simulink model "sim_punto4"  (R2021b)
settings: Solver=VariableStepAuto  StartTime=0.0  StopTime=10.0  RelTol=1e-3
values from neighbouring files (symbols this model uses):
  A = [0 1 0 0 0 0 0 0 0 0 0 0 ... (first row only)    [punto4.m]
  B = [0; 0; 0; 0; 0; 0; 0; 0; 0; 0; 0; 1]    [punto4.m]
  C = [1 0 0 0 0 0 0 0 0 0 0 0]    [punto4.m]
  C_states = eye(12)    [punto4.m]
  D_states = [0 0 0 0 0 0 0 0 0 0 0 0]'    [punto4.m]
  N3 = 27    [punto4.m]
  Q = [1+q 0 0 0 0 0 0 0 0 0 0 0 ... (first row only)    [punto4.m]
  R = r    (= 1e-05)    [punto4.m]
  S = [0 0 0 0 0 0 0 0 0 0 0 0 ... (first row only)    [punto4.m]
  Ts = 0.1    [punto4.m]
  U_max = 15    [punto4.m]
  U_min = -15    [punto4.m]
  Ubar = inv(g)*Ybar    [punto4.m]
  umax = 15    [punto4.m]
  umin = -15    [punto4.m]
  x0 = [0 0 0 0 0 0 0 0 0 0 0 0]    [punto4.m]
  Xbar = -inv(A) * B * Ubar    [punto4.m]
undefined symbols (not defined in the file or in its folder): mympc
settings Model: Creator=danie  LastModifiedBy=danie

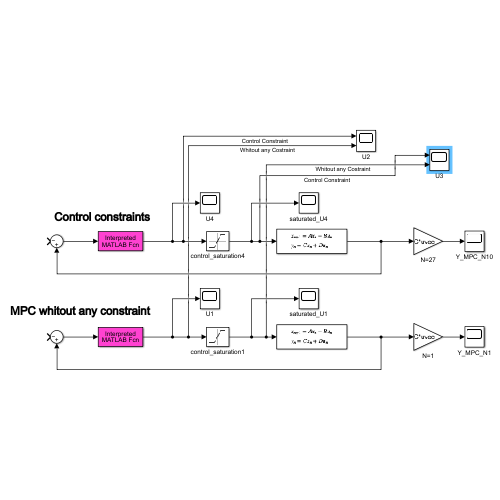
[thumbnail: Simulink's stored preview of the top-level diagram]
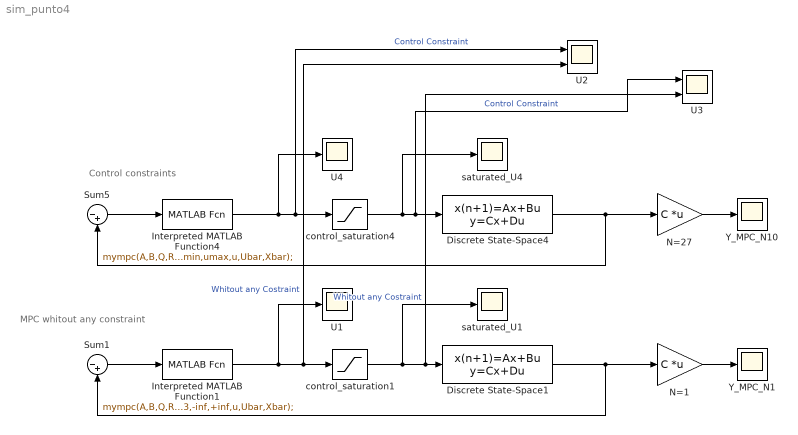
== system sim_punto4 ==
  note: Control constraints
  note: MPC whitout any constraint
  Discrete State-Space1 : DiscreteStateSpace  A=A  B=B  C=C_states  D=D_states  InitialCondition=x0  SampleTime=Ts
  Discrete State-Space4 : DiscreteStateSpace  A=A  B=B  C=C_states  D=D_states  InitialCondition=x0  SampleTime=Ts
  Interpreted MATLAB Function1 : MATLABFcn  MATLABFcn=mympc(A,B,Q,R,S,N3,-inf,+inf,u,Ubar,Xbar);  OutputDimensions=1
  Interpreted MATLAB Function4 : MATLABFcn  MATLABFcn=mympc(A,B,Q,R,S,N3,umin,umax,u,Ubar,Xbar);  OutputDimensions=1
  N=1 : Gain  Gain=C  Multiplication=Matrix(K*u) (u vector)
  N=27 : Gain  Gain=C  Multiplication=Matrix(K*u) (u vector)
  Sum1 : Sum  Inputs=|-+
  Sum5 : Sum  Inputs=|-+
  U1 : Scope
  U2 : Scope  NumInputPorts=2
  U3 : Scope  NumInputPorts=2
  U4 : Scope
  Y_MPC_N1 : Scope
  Y_MPC_N10 : Scope
  control_saturation1 : Saturate  UpperLimit=U_max  LowerLimit=U_min
  control_saturation4 : Saturate  UpperLimit=U_max  LowerLimit=U_min
  saturated_U1 : Scope
  saturated_U4 : Scope
  wires:
  Sum5/1 -> Interpreted MATLAB Function4/1
  Interpreted MATLAB Function4/1 -> U2/1, control_saturation4/1, U4/1  "Control Constraint"
  Discrete State-Space4/1 -> Sum5/2, N=27/1
  control_saturation4/1 -> saturated_U4/1, U3/1, Discrete State-Space4/1  "Control Constraint"
  N=27/1 -> Y_MPC_N10/1
  N=1/1 -> Y_MPC_N1/1
  Interpreted MATLAB Function1/1 -> U2/2, control_saturation1/1, U1/1  "Whitout any Costraint"
  control_saturation1/1 -> saturated_U1/1, U3/2, Discrete State-Space1/1  "Whitout any Costraint"
  Discrete State-Space1/1 -> Sum1/2, N=1/1
  Sum1/1 -> Interpreted MATLAB Function1/1
